simulink model "microgrid_ESS_Desktop"  (R2020b)
settings: Solver=FixedStepDiscrete  StartTime=0.0  StopTime=90  FixedStep=Ts  RelTol=1e-3
PreLoadFcn:
  | % Create Bus Object for Power Measurements
  | 
  | %Bus Object - Backup Power
  | BusElement(1) = Simulink.BusElement;
  | BusElement(1).Name = 'P';
  | BusElement(1).Dimensions = 1;
  | BusElement(1).DimensionsMode = 'Fixed';
  | BusElement(1).DataType = 'double';
  | BusElement(1).Complexity = 'real';
  | 
  | BusElement(2) = Simulink.BusElement;
  | BusElement(2).Name = 'Q';
  | BusElement(2).Dimensions = 1;
  | BusElement(2).DimensionsMode = 'Fixed';
  | BusElement(2).DataType = 'double';
  | BusElement(2).Complexity = 'real';
  | 
  | Batt = Simulink.Bus;
  | Batt.Elements = BusElement;
  | 
  | % Bus object - Grid Power
  | BusElement(1) = Simulink.BusElement;
  | BusElement(1).Name = 'P';
  | BusElement(1).Dimensions = 1;
  | BusElement(1).DimensionsMode = 'Fixed';
  | BusElement(1).DataType = 'double';
  | BusElement(1).Complexity = 'real';
  | 
  | BusElement(2) = Simulink.BusElement;
  | BusElement(2).Name = 'Q';
  | BusElement(2).Dimensions = 1;
  | BusElement(2).DimensionsMode = 'Fixed';
  | BusElement(2).DataType = 'double';
  | BusElement(2).Complexity = 'real';
  | 
  | Grid = Simulink.Bus;
  | Grid.Elements = BusElement;
  | 
  | % Bus object: PowerBus
  | BusElement(1) = Simulink.BusElement;
  | BusElement(1).Name = 'Grid';
  | BusElement(1).DataType = 'Bus: Grid';
  | 
  | BusElement(2) = Simulink.BusElement;
  | BusElement(2).Name = 'Batt';
  | BusElement(2).DataType = 'Bus: Batt';
  | 
  | PowerBus = Simulink.Bus;
  | PowerBus.Elements = BusElement;
  | clear BusElement
  | 
  | Batt_Mode = Simulink.Bus;
  | BusElement(1) = Simulink.BusElement;
  | BusElement(1).Name = 'CurrOrVoltSource';
  | BusElement(1).Complexity = 'real';
  | BusElement(1).Dimensions = 1;
  | BusElement(1).DataType = 'double';
  | BusElement(1).DimensionsMode = 'Fixed';
  | 
  | BusElement(2) = Simulink.BusElement;
  | BusElement(2).Name = 'GenOrSynchMode';
  | BusElement(2).Complexity = 'real';
  | BusElement(2).Dimensions = 1;
  | BusElement(2).DataType = 'double';
  | BusElement(2).DimensionsMode = 'Fixed';
  | 
  | Batt_Mode.Elements = BusElement;
  | 
  | ESS_Mode = Simulink.Bus;
  | BusElement(1) = Simulink.BusElement;
  | BusElement(1).Name = 'ControlType';
  | BusElement(1).Complexity = 'real';
  | BusElement(1).Dimensions = 1;
  | BusElement(1).DataType = 'double';
  | BusElement(1).DimensionsMode = 'Fixed';
  | 
  | BusElement(2) = Simulink.BusElement;
  | BusElement(2).Name = 'Batt_Mode';
  | BusElement(2).Complexity = 'real';
  | BusElement(2).Dimensions = 1;
  | BusElement(2).DataType = 'Bus: Batt_Mode';
  | BusElement(2).DimensionsMode = 'Fixed';
  | 
  | ESS_Mode.Elements = BusElement;
  | 
  | clear BusElement;
InitFcn:
  | %Ts = 1/(50*100);
  | %Tc = 0.01;
  | 
  | 
  | 
  | %Ts = 80e-6*2;
  | Ts = 200e-6;
  | Ts_Control=Ts;
  | Tc = Ts_Control;
  | Ts_PLC = Ts*500;
  | 
  | genMax = 50*100e3;
libraries: microgridLib x37, simulink x7, powerlib x6, powerlib_meascontrol x2
settings Model: SimulationMode=accelerator  Creator=jlesage  LastModifiedBy=jlesage

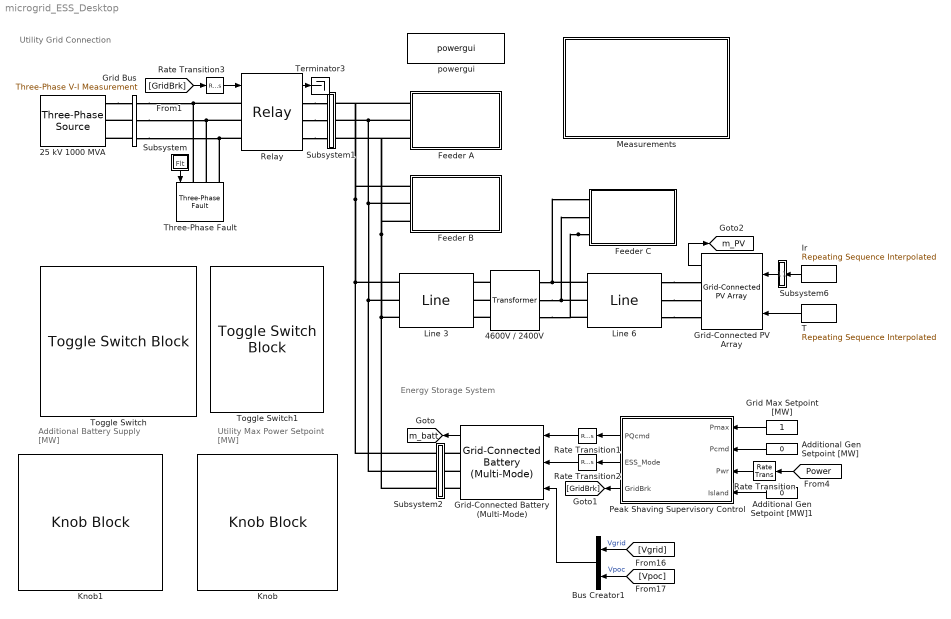
== system microgrid_ESS_Desktop ==
  note: Utility Grid Connection
  note: Utility Max Power
      | Setpoint [MW]
  note: Energy Storage System
  note: Additional Battery
      | Supply [MW]
  25 kV 1000 MVA : powerlib/Electrical Sources/Three-Phase Source  InternalConnection=Yg  VoltagePhases=off  Voltage=25e3  PhaseAngle=0.34499  Voltage_phases=[25e3 25e3 25e3]/sqrt(3)  PhaseAngles_phases=[0 -120 +120]  Frequency=60  NonIdealSource=on  SpecifyImpedance=on  Resistance=25^2/1000/10  Inductance=25^2/1000/377  ShortCircuitLevel=1000e6  BaseVoltage=25e3  XRratio=10  BusType=swing  Pref=0  Qref=0  Prefabc=[10e3, 10e3, 10e3]  Qrefabc=[0, 0, 0]  Qmin=-Inf  Qmax=Inf
  4600V / 2400V : microgridLib/Transformer  kS=5000  Freq=60  Vp=4600  Vs=2400  Zperc=6.37  Ratio=3.5
  Additional Gen Setpoint [MW] : Constant  Value=0
  Additional Gen Setpoint [MW]1 : Constant  Value=0
  Bus Creator1 : BusCreator  Inputs=2
  Feeder A : Subsystem
  Feeder B : Subsystem
  Feeder C : Subsystem
  Grid Bus : powerlib/Measurements/Three-Phase V-I Measurement  VoltageMeasurement=phase-to-ground  SetLabelV=on  LabelV=Vgrid  Vpu=off  VpuLL=off  CurrentMeasurement=yes  SetLabelI=on  LabelI=Igrid  Ipu=off  Pbase=100e6  Vbase=(25000)*1.00007  OutputType=Complex  PhasorSimulation=off  PSBequivalent=0
  Grid Max Setpoint [MW] : Constant
  Grid-Connected Battery (Multi-Mode) : microgridLib/Grid-Connected Battery (Multi-Mode)  Pmod=25  Vnom_dc=480  Bcap=500  Vnom_prim=4600  Fnom=60  Ts=Ts  Ts_Control=Ts_Control
  Grid-Connected PV Array : microgridLib/Grid-Connected PV Array  Pmod=5  Vnom_prim=2400  Fnom=60  Ts=Ts  Ts_Control=Ts_Control
  Ir : simulink/Sources/Repeating Sequence Interpolated  OutValues=[1000 920 950 800 950 875 1000]'  TimeValues=[0 5 10 25 30 45 60]'*1.1  LookUpMeth=Interpolation-Use End Values  tsamp=Ts  OutMin=[]  OutMax=[]  OutDataTypeStr=double  OutputDataTypeScalingMode=double  OutDataType=fixdt(0,8)  OutScaling=2^-10
  Knob : KnobBlock  ScaleMax=3
  Knob1 : KnobBlock  ScaleMin=-3  ScaleMax=3
  Line 3 : microgridLib/Line   gauge=500 Kcmil  Freq=60  Length_ft=300  Ratio=3
  Line 6 : microgridLib/Line   gauge=4/0 AWG  Freq=60  Length_ft=25  Ratio=3
  Measurements : Subsystem
  Peak Shaving Supervisory Control : Subsystem
  Rate Transition : RateTransition  OutPortSampleTime=Ts_PLC
  Rate Transition1 : RateTransition  OutPortSampleTime=Ts_Control
  Rate Transition2 : RateTransition  OutPortSampleTime=Ts_Control
  Rate Transition3 : RateTransition  InitialCondition=1  OutPortSampleTime=Ts
  Relay : microgridLib/Relay  SystemSampleTime=-1  VariantActivationTime=update diagram  Latency=0  AutoFrameSizeCalculation=off
  Subsystem : Subsystem
  Subsystem1 : Subsystem
  Subsystem2 : Subsystem
  Subsystem6 : Subsystem
  T : simulink/Sources/Repeating Sequence Interpolated  OutValues=[45 40 40 41 46 47 45]'  TimeValues=[0 5 10 25 30 45 60]'*1.25  LookUpMeth=Interpolation-Use End Values  tsamp=Ts  OutMin=[]  OutMax=[]  OutDataTypeStr=double  OutputDataTypeScalingMode=double  OutDataType=fixdt(0,8)  OutScaling=2^-10
  Terminator3 : Terminator
  Three-Phase Fault : powerlib/Elements/Three-Phase Fault  InitialStates=0  FaultA=on  FaultB=on  FaultC=on  GroundFault=on  SwitchTimes="[1/60  5/60]"  External=on  SwitchStatus=NaN  FaultResistance=0.01  GroundResistance=0.001  SnubberResistance=inf  SnubberCapacitance=inf  Measurements=None
  Toggle Switch : ToggleSwitchBlock  LabelPosition=Hide
      settings: Values={{'Grid Connect', 'Island'}, [0 1]}
  Toggle Switch1 : ToggleSwitchBlock  LabelPosition=Hide
      settings: Values={{'Clear', 'Cloud'}, [0 1]}
  powergui : powerlib/powergui  Priority=2  SimulationMode=Discrete  SampleTime=Ts  frequency=60  Iterations=50  frequencyindice=60  Pbase=1e6  ErrMax=0.0001  UnitsV=kV  UnitsW=MW  buscounter=6  FunctionMessages=off  echomessages=off  EnableUseOfTLC=off  CurrentSourceSwitches=off  DisableSnubberDevices=off  DisableRonSwitches=off  DisableVfSwitches=off  DisplayEquations=off  AutomaticDiscreteSolvers=off  SolverType=Tustin/Backward Euler (TBE)  Interpol=off  ExternalGateDelay=off  methode=off  Ts=0  x0status=blocks  SPID=off  SwTol=0  HookPort=off  NonlinearTolerance=1e-4  nMaxIteration=100  ContinueOnMaxIteration=off  RestoreLinks=warning  ResistiveCurrentMeasurement=off  Frange=logspace(0,3,50)  Ylog=off  Xlog=off  ShowGrid=off  save=off  variable=ZData  structure=0  ZoomFFT=on  StartTime=0.0  cycles=2  DisplayStyle=off  fundamental=60  FreqAxis=off  MaxFrequency=1000  frequencyindicesteady=1  RmsSteady=1  display=off
  tag scope: m_PV=global, m_batt=global
  wires:
  Grid-Connected Battery (Multi-Mode)/1 -> [m_batt]
  Additional Gen Setpoint [MW]1/1 -> Peak Shaving Supervisory Control/4(Island)
  T/1 -> Grid-Connected PV Array/2
  [Power] -> Rate Transition/1
  Additional Gen Setpoint [MW]/1 -> Peak Shaving Supervisory Control/2(Pcmd)
  Rate Transition/1 -> Peak Shaving Supervisory Control/3(Pwr)
  Rate Transition2/1 -> Grid-Connected Battery (Multi-Mode)/2
  Rate Transition3/1 -> Relay/1
  Ir/1 -> Subsystem6/1(In1)
  Subsystem/1(Flt) -> Three-Phase Fault/1
  Peak Shaving Supervisory Control/3(GridBrk) -> [GridBrk]
  Peak Shaving Supervisory Control/2(ESS_Mode) -> Rate Transition2/1
  Grid Max Setpoint [MW]/1 -> Peak Shaving Supervisory Control/1(Pmax)
  [GridBrk] -> Rate Transition3/1
  Bus Creator1/1 -> Grid-Connected Battery (Multi-Mode)/3
  [Vgrid] -> Bus Creator1/1  "Vgrid"
  Rate Transition1/1 -> Grid-Connected Battery (Multi-Mode)/1
  Grid-Connected PV Array/1 -> [m_PV]
  Peak Shaving Supervisory Control/1(PQcmd) -> Rate Transition1/1
  Relay/1 -> Terminator3/1
  [Vpoc] -> Bus Creator1/2  "Vpoc"
  Subsystem6/1(Out1) -> Grid-Connected PV Array/1
  connections:
  Line 3/LConn3 -- Feeder A/LConn3 -- Subsystem1/RConn3 -- Feeder B/LConn3 -- Subsystem2/LConn3
  Feeder B/LConn2 -- Subsystem1/RConn2 -- Feeder A/LConn2 -- Subsystem2/LConn2 -- Line 3/LConn2
  Line 3/LConn1 -- Feeder A/LConn1 -- Subsystem1/RConn1 -- Feeder B/LConn1 -- Subsystem2/LConn1
  Relay/LConn3 -- Grid Bus/RConn3 -- Three-Phase Fault/LConn3
  Line 6/LConn1 -- 4600V / 2400V/RConn1 -- Feeder C/LConn1
  Relay/LConn1 -- Grid Bus/RConn1 -- Three-Phase Fault/LConn1
  Line 6/LConn2 -- 4600V / 2400V/RConn2 -- Feeder C/LConn2
  Feeder C/LConn3 -- 4600V / 2400V/RConn3 -- Line 6/LConn3
  Relay/LConn2 -- Grid Bus/RConn2 -- Three-Phase Fault/LConn2
  25 kV 1000 MVA/RConn1 -- Grid Bus/LConn1
  4600V / 2400V/LConn3 -- Line 3/RConn3
  Grid-Connected Battery (Multi-Mode)/RConn2 -- Subsystem2/RConn2
  4600V / 2400V/LConn1 -- Line 3/RConn1
  Grid Bus/LConn3 -- 25 kV 1000 MVA/RConn3
  Relay/RConn3 -- Subsystem1/LConn3
  Relay/RConn2 -- Subsystem1/LConn2
  4600V / 2400V/LConn2 -- Line 3/RConn2
  Line 6/RConn1 -- Grid-Connected PV Array/RConn1
  Grid-Connected Battery (Multi-Mode)/RConn1 -- Subsystem2/RConn1
  Line 6/RConn2 -- Grid-Connected PV Array/RConn2
  Relay/RConn1 -- Subsystem1/LConn1
  Grid-Connected Battery (Multi-Mode)/RConn3 -- Subsystem2/RConn3
  Line 6/RConn3 -- Grid-Connected PV Array/RConn3
  Grid Bus/LConn2 -- 25 kV 1000 MVA/RConn2

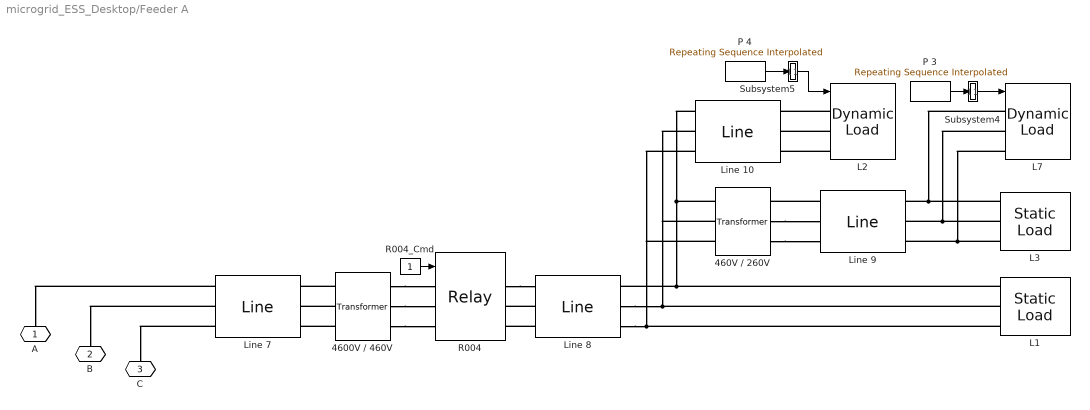
== system microgrid_ESS_Desktop/Feeder A ==
  4600V / 460V : microgridLib/Transformer  kS=5000  Freq=60  Vp=4600  Vs=460  Zperc=5.1  Ratio=2.5
  460V / 260V : microgridLib/Transformer  kS=2000  Freq=60  Vp=460  Vs=240  Zperc=5.1  Ratio=2.5
  L1 : microgridLib/Static Load  kS=25  PF=0.9  Vrms=460  Freq=60
  L2 : microgridLib/Dynamic Load  Vrms=460  Freq=60  Ts=Ts  Tau=1e-4
  L3 : microgridLib/Static Load  kS=25  PF=1  Vrms=240  Freq=60
  L7 : microgridLib/Dynamic Load  Vrms=240  Freq=60  Ts=Ts  Tau=1e-4
  Line 10 : microgridLib/Line   gauge=3/0 AWG  Freq=60  Length_ft=50  Ratio=3
  Line 7 : microgridLib/Line   gauge=500 Kcmil  Freq=60  Length_ft=500  Ratio=3
  Line 8 : microgridLib/Line   gauge=500 Kcmil  Freq=60  Length_ft=100  Ratio=3
  Line 9 : microgridLib/Line   gauge=1/0 AWG  Freq=60  Length_ft=25  Ratio=3
  P 3 : simulink/Sources/Repeating Sequence Interpolated  OutValues=[0 -1e5 3e5 10e5 0e5 5e5 0]'/50  TimeValues=[0 5 10 25 30 45 60]'*0.2  LookUpMeth=Interpolation-Use End Values  tsamp=Ts  OutMin=[]  OutMax=[]  OutDataTypeStr=double  OutputDataTypeScalingMode=double  OutDataType=fixdt(0,8)  OutScaling=2^-10
  P 4 : simulink/Sources/Repeating Sequence Interpolated  OutValues=[0 1e5 -3e5 10e5 0e5 5e5 0]'/75  TimeValues=[0 5 10 25 30 45 60]'*0.5  LookUpMeth=Interpolation-Use End Values  tsamp=Ts  OutMin=[]  OutMax=[]  OutDataTypeStr=double  OutputDataTypeScalingMode=double  OutDataType=fixdt(0,8)  OutScaling=2^-10
  R004 : microgridLib/Relay  SystemSampleTime=-1  VariantActivationTime=update diagram  Latency=0  AutoFrameSizeCalculation=off
  R004_Cmd : Constant
  Subsystem4 : Subsystem
  Subsystem5 : Subsystem
  A : PMIOPort  Side=Left
  B : PMIOPort  Port=2  Side=Left
  C : PMIOPort  Port=3  Side=Left
  wires:
  R004_Cmd/1 -> R004/1
  P 3/1 -> Subsystem4/1(In1)
  Subsystem4/1(Out1) -> L7/1
  P 4/1 -> Subsystem5/1(In1)
  Subsystem5/1(Out1) -> L2/1
  connections:
  Line 7/LConn2 -- B/RConn1
  Line 7/LConn3 -- C/RConn1
  Line 7/LConn1 -- A/RConn1
  4600V / 460V/RConn1 -- R004/LConn1
  4600V / 460V/LConn3 -- Line 7/RConn3
  Line 8/RConn3 -- 460V / 260V/LConn3 -- Line 10/LConn3 -- L1/LConn3
  L2/LConn1 -- Line 10/RConn1
  R004/RConn1 -- Line 8/LConn1
  4600V / 460V/RConn3 -- R004/LConn3
  Line 8/LConn3 -- R004/RConn3
  Line 8/LConn2 -- R004/RConn2
  4600V / 460V/LConn1 -- Line 7/RConn1
  Line 10/LConn1 -- 460V / 260V/LConn1 -- L1/LConn1 -- Line 8/RConn1
  Line 8/RConn2 -- 460V / 260V/LConn2 -- Line 10/LConn2 -- L1/LConn2
  4600V / 460V/LConn2 -- Line 7/RConn2
  4600V / 460V/RConn2 -- R004/LConn2
  L3/LConn3 -- L7/LConn3 -- Line 9/LConn3
  L2/LConn2 -- Line 10/RConn2
  L2/LConn3 -- Line 10/RConn3
  460V / 260V/RConn2 -- Line 9/RConn2
  Line 9/RConn1 -- 460V / 260V/RConn1
  L3/LConn1 -- L7/LConn1 -- Line 9/LConn1
  460V / 260V/RConn3 -- Line 9/RConn3
  L3/LConn2 -- L7/LConn2 -- Line 9/LConn2

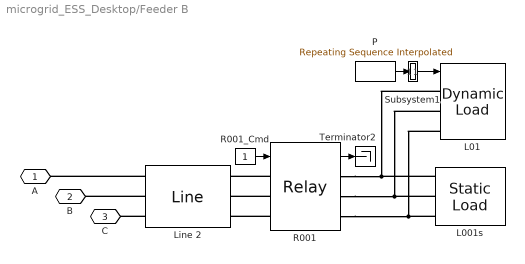
== system microgrid_ESS_Desktop/Feeder B ==
  L001s : microgridLib/Static Load  kS=700  PF=0.99  Vrms=4600  Freq=60
  L01 : microgridLib/Dynamic Load  Vrms=4600  Freq=60  Ts=Ts  Tau=1e-4
  Line 2 : microgridLib/Line   gauge=500 Kcmil  Freq=60  Length_ft=100  Ratio=3
  "P " : simulink/Sources/Repeating Sequence Interpolated  OutValues=[0 -1e5 3e5 10e5 0e5 9e5 0 2e5 -1e5 8e5 6e5 0e5]'*0.75  TimeValues=[0 5 10 25 30 45 55 60 65 70 80 90]'  LookUpMeth=Interpolation-Use End Values  tsamp=Ts  OutMin=[]  OutMax=[]  OutDataTypeStr=double  OutputDataTypeScalingMode=double  OutDataType=fixdt(0,8)  OutScaling=2^-10
  R001 : microgridLib/Relay  SystemSampleTime=-1  VariantActivationTime=update diagram  Latency=0  AutoFrameSizeCalculation=off
  R001_Cmd : Constant
  Subsystem1 : Subsystem
  Terminator2 : Terminator
  A : PMIOPort  Side=Left
  B : PMIOPort  Port=2  Side=Left
  C : PMIOPort  Port=3  Side=Left
  wires:
  R001/1 -> Terminator2/1
  Subsystem1/1(Out1) -> L01/1
  R001_Cmd/1 -> R001/1
  "P "/1 -> Subsystem1/1(In1)
  connections:
  Line 2/LConn1 -- A/RConn1
  Line 2/LConn3 -- C/RConn1
  Line 2/LConn2 -- B/RConn1
  R001/LConn1 -- Line 2/RConn1
  R001/RConn2 -- L01/LConn2 -- L001s/LConn2
  R001/RConn1 -- L001s/LConn1 -- L01/LConn1
  R001/LConn3 -- Line 2/RConn3
  R001/RConn3 -- L01/LConn3 -- L001s/LConn3
  R001/LConn2 -- Line 2/RConn2

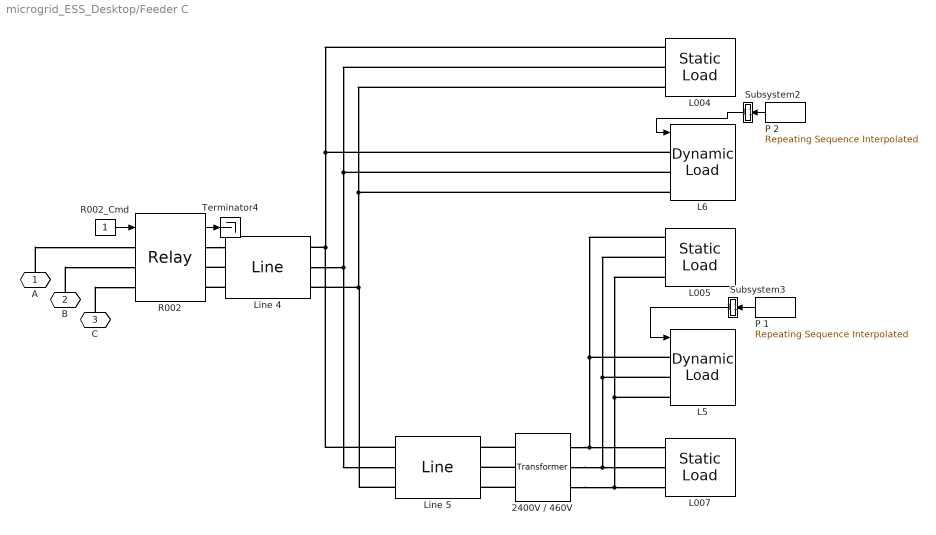
== system microgrid_ESS_Desktop/Feeder C ==
  2400V / 460V : microgridLib/Transformer  kS=2000  Freq=60  Vp=2400  Vs=460  Zperc=5.18  Ratio=2.5
  L004 : microgridLib/Static Load  kS=25  PF=0.9  Vrms=2400  Freq=60
  L005 : microgridLib/Static Load  kS=25  PF=0.8  Vrms=460  Freq=60
  L007 : microgridLib/Static Load  kS=115  PF=0.9  Vrms=460  Freq=60
  L5 : microgridLib/Dynamic Load  Vrms=460  Freq=60  Ts=Ts  Tau=1e-4
  L6 : microgridLib/Dynamic Load  Vrms=2400  Freq=60  Ts=Ts  Tau=1e-4
  Line 4 : microgridLib/Line   gauge=500 Kcmil  Freq=60  Length_ft=100  Ratio=3
  Line 5 : microgridLib/Line   gauge=4/0 AWG  Freq=60  Length_ft=250  Ratio=3
  P 1 : simulink/Sources/Repeating Sequence Interpolated  OutValues=[0 1e5 -3e5 10e5 0e5 5e5 0]'/100  TimeValues=[0 5 10 25 30 45 60]'*0.9  LookUpMeth=Interpolation-Use End Values  tsamp=Ts  OutMin=[]  OutMax=[]  OutDataTypeStr=double  OutputDataTypeScalingMode=double  OutDataType=fixdt(0,8)  OutScaling=2^-10
  P 2 : simulink/Sources/Repeating Sequence Interpolated  OutValues=[0 -1e5 3e5 10e5 0e5 5e5 0]'/10  TimeValues=[0 5 10 25 30 45 60]'*0.1  LookUpMeth=Interpolation-Use End Values  tsamp=Ts  OutMin=[]  OutMax=[]  OutDataTypeStr=double  OutputDataTypeScalingMode=double  OutDataType=fixdt(0,8)  OutScaling=2^-10
  R002 : microgridLib/Relay  SystemSampleTime=-1  VariantActivationTime=update diagram  Latency=0  AutoFrameSizeCalculation=off
  R002_Cmd : Constant
  Subsystem2 : Subsystem
  Subsystem3 : Subsystem
  Terminator4 : Terminator
  A : PMIOPort  Side=Left
  B : PMIOPort  Port=2  Side=Left
  C : PMIOPort  Port=3  Side=Left
  wires:
  R002_Cmd/1 -> R002/1
  R002/1 -> Terminator4/1
  Subsystem3/1(Out1) -> L5/1
  Subsystem2/1(Out1) -> L6/1
  P 1/1 -> Subsystem3/1(In1)
  P 2/1 -> Subsystem2/1(In1)
  connections:
  A/RConn1 -- R002/LConn1
  B/RConn1 -- R002/LConn2
  C/RConn1 -- R002/LConn3
  Line 4/LConn3 -- R002/RConn3
  Line 5/LConn1 -- L6/LConn1 -- L004/LConn1 -- Line 4/RConn1
  2400V / 460V/LConn3 -- Line 5/RConn3
  L005/LConn2 -- L5/LConn2 -- 2400V / 460V/RConn2 -- L007/LConn2
  Line 4/LConn2 -- R002/RConn2
  2400V / 460V/LConn1 -- Line 5/RConn1
  R002/RConn1 -- Line 4/LConn1
  2400V / 460V/LConn2 -- Line 5/RConn2
  L005/LConn3 -- L5/LConn3 -- 2400V / 460V/RConn3 -- L007/LConn3
  L005/LConn1 -- L5/LConn1 -- 2400V / 460V/RConn1 -- L007/LConn1
  Line 4/RConn2 -- L6/LConn2 -- L004/LConn2 -- Line 5/LConn2
  Line 5/LConn3 -- L6/LConn3 -- L004/LConn3 -- Line 4/RConn3

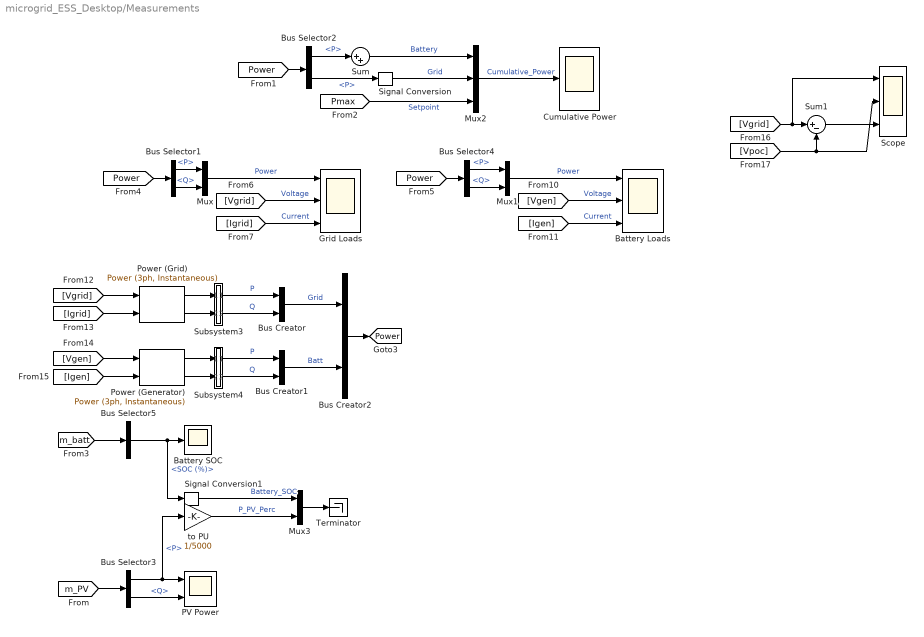
== system microgrid_ESS_Desktop/Measurements ==
  Battery Loads : Scope  NumInputPorts=3
  Battery SOC : Scope
  Bus Creator : BusCreator  Inputs=2
  Bus Creator1 : BusCreator  Inputs=2
  Bus Creator2 : BusCreator  Inputs=2
  Bus Selector1 : BusSelector  OutputSignals=Grid.P,Grid.Q
  Bus Selector2 : BusSelector  OutputSignals=Batt.P,Grid.P
  Bus Selector3 : BusSelector  OutputSignals=Grid.P,Grid.Q
  Bus Selector4 : BusSelector  OutputSignals=Batt.P,Batt.Q
  Bus Selector5 : BusSelector  OutputSignals=Battery.SOC (%)
  Cumulative Power : Scope
  Grid Loads : Scope  NumInputPorts=3
  Mux : Mux  Inputs=2
  Mux1 : Mux  Inputs=2
  Mux2 : Mux  Inputs=3
  Mux3 : Mux  Inputs=2
  PV Power : Scope  NumInputPorts=2
  Power (Generator) : powerlib_meascontrol/Measurements/Power (3ph, Instantaneous)
  Power (Grid) : powerlib_meascontrol/Measurements/Power (3ph, Instantaneous)
  Scope : Scope  NumInputPorts=3
  Signal Conversion : SignalConversion  OverrideOpt=off
  Signal Conversion1 : SignalConversion  OverrideOpt=off
  Subsystem3 : Subsystem
  Subsystem4 : Subsystem
  Sum : Sum  Inputs=|++
  Sum1 : Sum  Inputs=|+-
  Terminator : Terminator
  to PU : Gain  Gain=1/5000
  tag scope: Power=global
  wires:
  Bus Selector1/1 -> Mux/1  "<P>"
  Bus Selector1/2 -> Mux/2  "<Q>"
  Mux/1 -> Grid Loads/1  "Power"
  [Vgrid] -> Grid Loads/2  "Voltage"
  [Igrid] -> Grid Loads/3  "Current"
  Bus Selector4/1 -> Mux1/1  "<P>"
  Bus Selector4/2 -> Mux1/2  "<Q>"
  Mux1/1 -> Battery Loads/1  "Power"
  [Vgen] -> Battery Loads/2  "Voltage"
  [Igen] -> Battery Loads/3  "Current"
  [Vgrid] -> Power (Grid)/1
  [Igrid] -> Power (Grid)/2
  [Vgen] -> Power (Generator)/1
  [Igen] -> Power (Generator)/2
  Bus Creator/1 -> Bus Creator2/1  "Grid"
  Bus Creator1/1 -> Bus Creator2/2  "Batt"
  Bus Creator2/1 -> [Power]
  [Power] -> Bus Selector1/1
  [Power] -> Bus Selector4/1
  Mux2/1 -> Cumulative Power/1  "Cumulative_Power"
  [Power] -> Bus Selector2/1
  [Pmax] -> Mux2/3  "Setpoint"
  Bus Selector2/1 -> Sum/1  "<P>"
  Bus Selector2/2 -> Signal Conversion/1  "<P>"
  Sum/1 -> Mux2/1  "Battery"
  Signal Conversion/1 -> Mux2/2  "Grid"
  [Vgrid] -> Scope/1, Sum1/1
  [Vpoc] -> Scope/2, Sum1/2
  Sum1/1 -> Scope/3
  Power (Grid)/1 -> Subsystem3/1(In1)
  Power (Grid)/2 -> Subsystem3/2(In2)
  Subsystem3/1(Out1) -> Bus Creator/1  "P"
  Subsystem3/2(Out2) -> Bus Creator/2  "Q"
  Power (Generator)/1 -> Subsystem4/1(In1)
  Power (Generator)/2 -> Subsystem4/2(In2)
  Subsystem4/1(Out1) -> Bus Creator1/1  "P"
  Subsystem4/2(Out2) -> Bus Creator1/2  "Q"
  [m_PV] -> Bus Selector3/1
  Bus Selector3/1 -> to PU/1, PV Power/1  "<P>"
  Bus Selector3/2 -> PV Power/2  "<Q>"
  [m_batt] -> Bus Selector5/1
  Bus Selector5/1 -> Signal Conversion1/1, Battery SOC/1  "<SOC (%)>"
  Mux3/1 -> Terminator/1
  to PU/1 -> Mux3/2  "P_PV_Perc"
  Signal Conversion1/1 -> Mux3/1  "Battery_SOC"

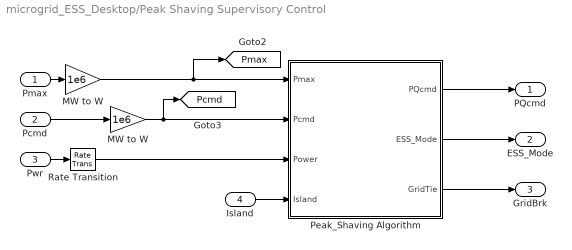
== system microgrid_ESS_Desktop/Peak Shaving Supervisory Control ==
  Pmax : Inport
  Pcmd : Inport  Port=2
  Pwr : Inport  Port=3
  Island : Inport  Port=4
  MW to W : Gain  Gain=1e6
  "MW to W " : Gain  Gain=1e6
  Peak_Shaving Algorithm : Stateflow chart  TreatAsAtomicUnit=on  SystemSampleTime=Ts_PLC
  Rate Transition : RateTransition  OutPortSampleTime=Ts_PLC
  PQcmd : Outport  SampleTime=Ts_PLC
  ESS_Mode : Outport  Port=2  SampleTime=Ts_PLC
  GridBrk : Outport  Port=3  SampleTime=Ts_PLC
  tag scope: Pcmd=global, Pmax=global
  wires:
  Rate Transition/1 -> Peak_Shaving Algorithm/3(Power)
  Pcmd/1 -> "MW to W "/1
  Pmax/1 -> MW to W/1
  Peak_Shaving Algorithm/1(PQcmd) -> PQcmd/1
  Pwr/1 -> Rate Transition/1
  "MW to W "/1 -> Peak_Shaving Algorithm/2(Pcmd), [Pcmd]
  MW to W/1 -> Peak_Shaving Algorithm/1(Pmax), [Pmax]
  Peak_Shaving Algorithm/3(GridTie) -> GridBrk/1
  Peak_Shaving Algorithm/2(ESS_Mode) -> ESS_Mode/1
  Island/1 -> Peak_Shaving Algorithm/4(Island)

== system microgrid_ESS_Desktop/Subsystem ==
  Fault : Constant  Value=0
  Triggered Subsystem : Subsystem  TreatAsAtomicUnit=on
  Flt : Outport
  wires:
  Fault/1 -> Triggered Subsystem/Enable
  Triggered Subsystem/1(Out1) -> Flt/1

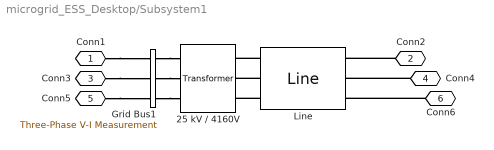
== system microgrid_ESS_Desktop/Subsystem1 ==
  "25 kV / 4160V " : microgridLib/Transformer  kS=6000  Freq=60  Vp=25e3  Vs=4600  Zperc=5.18  Ratio=2.5
  Grid Bus1 : powerlib/Measurements/Three-Phase V-I Measurement  VoltageMeasurement=phase-to-ground  SetLabelV=on  LabelV=Vpoc  Vpu=off  VpuLL=off  CurrentMeasurement=yes  SetLabelI=on  LabelI=Ipoc  Ipu=off  Pbase=100e6  Vbase=(25000)*1.00007  OutputType=Complex  PhasorSimulation=off  PSBequivalent=0
  "Line " : microgridLib/Line   gauge=500 Kcmil  Freq=60  Length_ft=100  Ratio=3
  Conn1 : PMIOPort  Side=Left
  Conn2 : PMIOPort  Port=2  Side=Right
  Conn3 : PMIOPort  Port=3  Side=Left
  Conn4 : PMIOPort  Port=4  Side=Right
  Conn5 : PMIOPort  Port=5  Side=Left
  Conn6 : PMIOPort  Port=6  Side=Right
  connections:
  Conn4/RConn1 -- "Line "/RConn2
  Conn6/RConn1 -- "Line "/RConn3
  Conn2/RConn1 -- "Line "/RConn1
  Conn3/RConn1 -- Grid Bus1/LConn2
  Conn1/RConn1 -- Grid Bus1/LConn1
  Conn5/RConn1 -- Grid Bus1/LConn3
  "Line "/LConn2 -- "25 kV / 4160V "/RConn2
  Grid Bus1/RConn1 -- "25 kV / 4160V "/LConn1
  Grid Bus1/RConn3 -- "25 kV / 4160V "/LConn3
  "Line "/LConn1 -- "25 kV / 4160V "/RConn1
  "Line "/LConn3 -- "25 kV / 4160V "/RConn3
  Grid Bus1/RConn2 -- "25 kV / 4160V "/LConn2

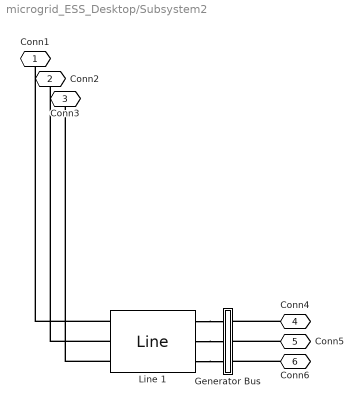
== system microgrid_ESS_Desktop/Subsystem2 ==
  Generator Bus : Subsystem
  Line 1 : microgridLib/Line   gauge=500 Kcmil  Freq=60  Length_ft=50  Ratio=3
  Conn1 : PMIOPort  Side=Left
  Conn2 : PMIOPort  Port=2  Side=Left
  Conn3 : PMIOPort  Port=3  Side=Left
  Conn4 : PMIOPort  Port=4  Side=Right
  Conn5 : PMIOPort  Port=5  Side=Right
  Conn6 : PMIOPort  Port=6  Side=Right
  connections:
  Line 1/LConn2 -- Conn2/RConn1
  Line 1/LConn1 -- Conn1/RConn1
  Conn4/RConn1 -- Generator Bus/LConn1
  Conn5/RConn1 -- Generator Bus/LConn2
  Conn6/RConn1 -- Generator Bus/LConn3
  Line 1/LConn3 -- Conn3/RConn1
  Line 1/RConn3 -- Generator Bus/RConn3
  Line 1/RConn2 -- Generator Bus/RConn2
  Line 1/RConn1 -- Generator Bus/RConn1

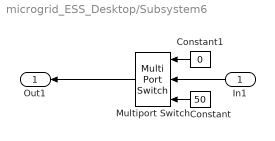
== system microgrid_ESS_Desktop/Subsystem6 ==
  In1 : Inport
  Constant : Constant  Value=50
  Constant1 : Constant  Value=0
  Multiport Switch : MultiPortSwitch  DataPortOrder=Zero-based contiguous  Inputs=2  zeroidx=on
  Out1 : Outport
  wires:
  Constant1/1 -> Multiport Switch/1
  Constant/1 -> Multiport Switch/3
  In1/1 -> Multiport Switch/2
  Multiport Switch/1 -> Out1/1

== system microgrid_ESS_Desktop/Feeder A/Subsystem4 ==
  In1 : Inport
  Mux : Mux  Inputs=2
  Q : Constant  Value=0
  Out1 : Outport
  wires:
  Mux/1 -> Out1/1
  Q/1 -> Mux/2
  In1/1 -> Mux/1

== system microgrid_ESS_Desktop/Feeder A/Subsystem5 ==
  In1 : Inport
  Mux : Mux  Inputs=2
  Q : Constant  Value=0
  Out1 : Outport
  wires:
  In1/1 -> Mux/1
  Q/1 -> Mux/2
  Mux/1 -> Out1/1

== system microgrid_ESS_Desktop/Feeder B/Subsystem1 ==
  In1 : Inport
  Mux : Mux  Inputs=2
  Q : Constant  Value=0
  Out1 : Outport
  wires:
  In1/1 -> Mux/1
  Q/1 -> Mux/2
  Mux/1 -> Out1/1

== system microgrid_ESS_Desktop/Feeder C/Subsystem2 ==
  In1 : Inport
  Mux : Mux  Inputs=2
  Q : Constant  Value=0
  Out1 : Outport
  wires:
  In1/1 -> Mux/1
  Q/1 -> Mux/2
  Mux/1 -> Out1/1

== system microgrid_ESS_Desktop/Feeder C/Subsystem3 ==
  In1 : Inport
  Mux : Mux  Inputs=2
  Q : Constant  Value=0
  Out1 : Outport
  wires:
  In1/1 -> Mux/1
  Q/1 -> Mux/2
  Mux/1 -> Out1/1

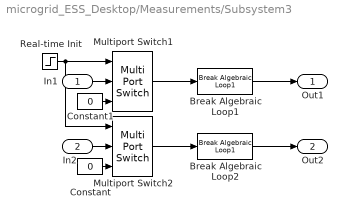
== system microgrid_ESS_Desktop/Measurements/Subsystem3 ==
  In1 : Inport
  In2 : Inport  Port=2
  Break Algebraic Loop1 : microgridLib/Dynamic Load/Calculate Current/Break Algebraic Loop1  Tau=0.01  Ts=Ts
  Break Algebraic Loop2 : microgridLib/Dynamic Load/Calculate Current/Break Algebraic Loop1  Tau=0.01  Ts=Ts
  Constant : Constant  Value=0
  Constant1 : Constant  Value=0
  Multiport Switch1 : MultiPortSwitch  DataPortOrder=Zero-based contiguous  Inputs=2  zeroidx=on
  Multiport Switch2 : MultiPortSwitch  DataPortOrder=Zero-based contiguous  Inputs=2  zeroidx=on
  Real-time Init : Step  Time=2  Before=1  After=0  SampleTime=Ts
  Out1 : Outport
  Out2 : Outport  Port=2
  wires:
  Real-time Init/1 -> Multiport Switch1/1, Multiport Switch2/1
  Constant1/1 -> Multiport Switch1/3
  Constant/1 -> Multiport Switch2/3
  Multiport Switch1/1 -> Break Algebraic Loop1/1
  In2/1 -> Multiport Switch2/2
  In1/1 -> Multiport Switch1/2
  Multiport Switch2/1 -> Break Algebraic Loop2/1
  Break Algebraic Loop1/1 -> Out1/1
  Break Algebraic Loop2/1 -> Out2/1

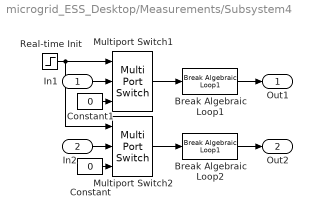
== system microgrid_ESS_Desktop/Measurements/Subsystem4 ==
  In1 : Inport
  In2 : Inport  Port=2
  Break Algebraic Loop1 : microgridLib/Dynamic Load/Calculate Current/Break Algebraic Loop1  Tau=0.01  Ts=Ts
  Break Algebraic Loop2 : microgridLib/Dynamic Load/Calculate Current/Break Algebraic Loop1  Tau=0.01  Ts=Ts
  Constant : Constant  Value=0
  Constant1 : Constant  Value=0
  Multiport Switch1 : MultiPortSwitch  DataPortOrder=Zero-based contiguous  Inputs=2  zeroidx=on
  Multiport Switch2 : MultiPortSwitch  DataPortOrder=Zero-based contiguous  Inputs=2  zeroidx=on
  Real-time Init : Step  Time=2  Before=1  After=0  SampleTime=Ts
  Out1 : Outport
  Out2 : Outport  Port=2
  wires:
  Multiport Switch2/1 -> Break Algebraic Loop2/1
  In1/1 -> Multiport Switch1/2
  In2/1 -> Multiport Switch2/2
  Multiport Switch1/1 -> Break Algebraic Loop1/1
  Constant/1 -> Multiport Switch2/3
  Constant1/1 -> Multiport Switch1/3
  Real-time Init/1 -> Multiport Switch2/1, Multiport Switch1/1
  Break Algebraic Loop1/1 -> Out1/1
  Break Algebraic Loop2/1 -> Out2/1

== system microgrid_ESS_Desktop/Subsystem/Triggered Subsystem ==
  Enable : EnablePort  StatesWhenEnabling=reset
  Constant : Constant  Value=0
  Delay : Delay  DelayLength=round(1.05*Ts_PLC/Ts)  InitialCondition=1
  Out1 : Outport  InitialOutput=0
  wires:
  Delay/1 -> Out1/1
  Constant/1 -> Delay/1

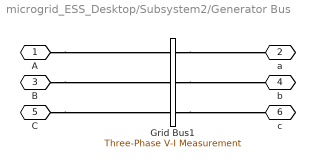
== system microgrid_ESS_Desktop/Subsystem2/Generator Bus ==
  Grid Bus1 : powerlib/Measurements/Three-Phase V-I Measurement  VoltageMeasurement=phase-to-ground  SetLabelV=on  LabelV=Vgen  Vpu=off  VpuLL=off  CurrentMeasurement=yes  SetLabelI=on  LabelI=Igen  Ipu=off  Pbase=100e6  Vbase=(25000)*1.00007  OutputType=Complex  PhasorSimulation=off  PSBequivalent=0
  A : PMIOPort  Side=Left
  a : PMIOPort  Port=2  Side=Right
  B : PMIOPort  Port=3  Side=Left
  b : PMIOPort  Port=4  Side=Right
  C : PMIOPort  Port=5  Side=Left
  c : PMIOPort  Port=6  Side=Right
  connections:
  Grid Bus1/RConn1 -- a/RConn1
  Grid Bus1/RConn2 -- b/RConn1
  Grid Bus1/RConn3 -- c/RConn1
  C/RConn1 -- Grid Bus1/LConn3
  B/RConn1 -- Grid Bus1/LConn2
  A/RConn1 -- Grid Bus1/LConn1

== stateflow chart microgrid_ESS_Desktop/Peak Shaving Supervisory Control/Peak_Shaving Algorithm ==
  state ESS_Control [parallel]
    during:
    P_Excess = Power.Grid.P + Power.Batt.P + Pcmd - Pmax;
    P_Max = genMax - Power.Batt.P;
    settings: executionOrder=1
    state GridConnected
      entry,during:
      ESS_Mode.ControlType = 0; %PQ Mode
      ESS_Mode.Batt_Mode.CurrOrVoltSource = 0; %Current Source
      isIsland = 0;
      state PeakShaving
        state MaxLocalGeneration
          during:
          PQcmd = [P_Max;0];
        state LoadFollowing
          during:
          PQcmd = [P_Excess;0];
        (default) -> LoadFollowing
        MaxLocalGeneration -> LoadFollowing : [Power.Batt.P < 0.95*genMax]
        LoadFollowing -> MaxLocalGeneration : [Power.Batt.P > genMax]
      state Nominal
        entry,during:
        PQcmd = [Pcmd;0];
      Nominal -> PeakShaving : [Power.Grid.P + Pcmd ...
          |  > Pmax]
      PeakShaving -> Nominal : [Power.Batt.P < 0 ...
          | && after(1,sec)]
      (default) -> Nominal
    state PrepareToIsland
      entry,during:
      PQcmd = [Power.Grid.P + Power.Batt.P + Pcmd; 0];
    state Islanded
      during:
      ESS_Mode.Batt_Mode.CurrOrVoltSource = 1; %Voltage Source
      ESS_Mode.Batt_Mode.GenOrSynchMode = 0; % No synch
      ESS_Mode.ControlType = 2; %No Current Control
    state Synchronize
      entry,during:
      ESS_Mode.Batt_Mode.CurrOrVoltSource = 1; %Voltage Source
      ESS_Mode.Batt_Mode.GenOrSynchMode = 1; % Synchronize
    (default) -> GridConnected
    GridConnected -> PrepareToIsland : [Island == 1]
    ESS_Control.Synchronize -> GridConnected : Reconnect
    PrepareToIsland -> ESS_Control.Islanded : [Power.Grid.P < 100]{isIsland = 1;}
    ESS_Control.Islanded -> ESS_Control.Synchronize : Synchronize
  state GridBreakerLogic [parallel]
    settings: executionOrder=2
    state Islanded
      during:
      GridTie = 0;
    state GridTied
      entry,during:
      GridTie = 1;
    state Reconnect
      entry,during:
      GridTie = 1;
      isIsland = 0;
    state Synchronize
    (default) -> GridTied
    GridTied -> GridBreakerLogic.Islanded : [isIsland == 1]
    Reconnect -> GridTied : [after(1,sec)] {send(Reconnect,ESS_Control)}
    GridBreakerLogic.Islanded -> GridBreakerLogic.Synchronize : [after(1,sec) && Island == 0] {send(Synchronize,ESS_Control)}
    GridBreakerLogic.Synchronize -> Reconnect : [after(2,sec)]
  data: Pmax input; genMax parameter; Pcmd input; Power input Bus: PowerBus; PQcmd output; ESS_Mode output Bus: ESS_Mode =0; GridTie output; P_Excess local; P_Max local; Island input; isIsland local
  events: Reconnect local FUNCTION_CALL_EVENT; Synchronize local FUNCTION_CALL_EVENT
